simulink model "single_wheel_translation"  (R2024b)
settings: Solver=ode1be  StartTime=t_0  StopTime=t_f  FixedStep=dt  RelTol=1e-5
undefined symbols (not defined in the file): final_torque, grav, initial_torque, step_time, vehicle_mass
settings Model: Creator=Yevgeniy Gorbachev  LastModifiedBy=yevge
settings SolverCC: ZeroCrossControl=DisableAll  ZeroCrossAlgorithm=Adaptive
settings DataIOCC: DatasetSignalFormat=timetable
settings RTWCC: GPUComputeCapability=3.5

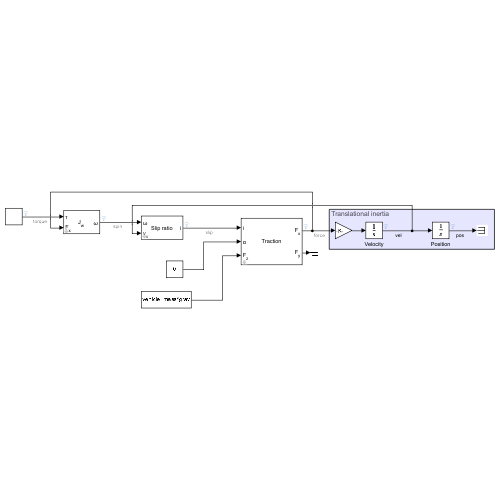
[thumbnail: Simulink's stored preview of the top-level diagram]
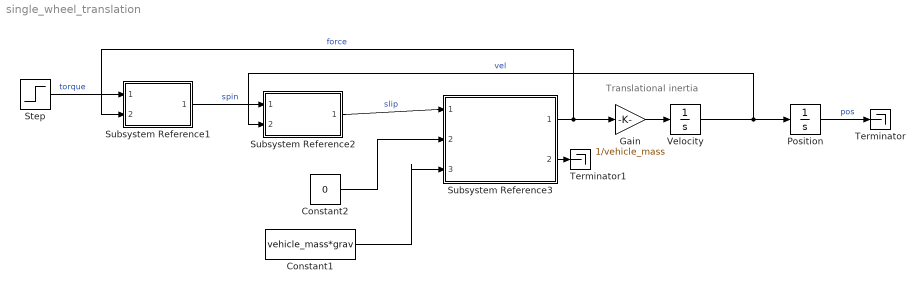
== system single_wheel_translation ==
  note: Translational inertia
  Constant1 : Constant  Value=vehicle_mass*grav
  Constant2 : Constant  Value=0
  Gain : Gain  Gain=1/vehicle_mass
  Position : Integrator
  Step : Step  Time=step_time  Before=initial_torque  After=final_torque  SampleTime=0
  Subsystem Reference1 : Subsystem  ReferencedSubsystem=wheel_inertia  radius=wheel_radius  spin_inertia=wheel_inertia  initial_spin=initial_spin
  Subsystem Reference2 : Subsystem  ReferencedSubsystem=slip_model  radius=wheel_radius  min_velocity=min_velocity
  Subsystem Reference3 : Subsystem  ReferencedSubsystem=traction
  Terminator : Terminator
  Terminator1 : Terminator
  Velocity : Integrator
  wires:
  Velocity/1 -> Subsystem Reference2/2, Position/1  "vel"
  Gain/1 -> Velocity/1
  Position/1 -> Terminator/1  "pos"
  Subsystem Reference1/1 -> Subsystem Reference2/1  "spin"
  Constant1/1 -> Subsystem Reference3/3
  Subsystem Reference2/1 -> Subsystem Reference3/1  "slip"
  Constant2/1 -> Subsystem Reference3/2
  Subsystem Reference3/2 -> Terminator1/1
  Subsystem Reference3/1 -> Subsystem Reference1/2, Gain/1  "force"
  Step/1 -> Subsystem Reference1/1  "torque"
